simulink subsystem "body_lift_compoenent"  (R2026a)
settings: Solver=VariableStepAuto
settings Model: Creator=joedo  LastModifiedBy=trist

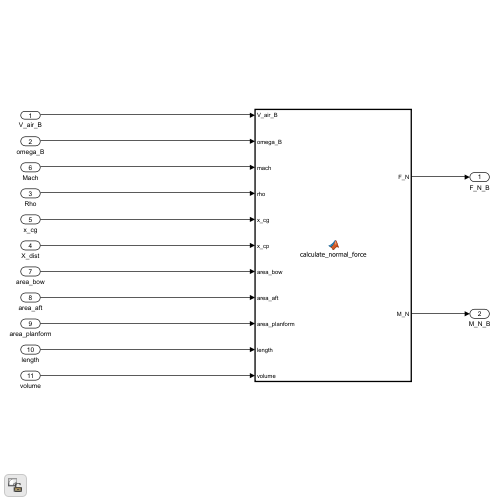
[thumbnail: Simulink's stored preview of the top-level diagram]
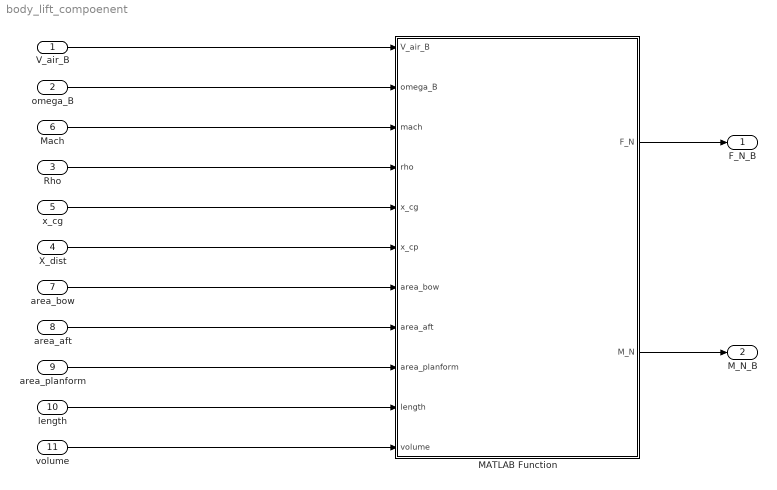
== system body_lift_compoenent ==
  "V_air_B " : Inport
  omega_B : Inport  Port=2
  Rho : Inport  Port=3
  X_dist : Inport  Port=4
  x_cg : Inport  Port=5
  Mach : Inport  Port=6
  area_bow : Inport  Port=7
  area_aft : Inport  Port=8
  area_planform : Inport  Port=9
  length : Inport  Port=10
  volume : Inport  Port=11
  MATLAB Function : MATLAB Function  TreatAsAtomicUnit=on
  F_N_B : Outport  VectorParamsAs1DForOutWhenUnconnected=off
  M_N_B : Outport  Port=2  VectorParamsAs1DForOutWhenUnconnected=off
  wires:
  X_dist/1 -> MATLAB Function/6(x_cp)
  Rho/1 -> MATLAB Function/4(rho)
  "V_air_B "/1 -> MATLAB Function/1(V_air_B)
  omega_B/1 -> MATLAB Function/2(omega_B)
  MATLAB Function/1(F_N) -> F_N_B/1
  MATLAB Function/2(M_N) -> M_N_B/1
  x_cg/1 -> MATLAB Function/5(x_cg)
  Mach/1 -> MATLAB Function/3(mach)
  area_bow/1 -> MATLAB Function/7(area_bow)
  area_aft/1 -> MATLAB Function/8(area_aft)
  area_planform/1 -> MATLAB Function/9(area_planform)
  length/1 -> MATLAB Function/10(length)
  volume/1 -> MATLAB Function/11(volume)

== matlab function body_lift_compoenent/MATLAB Function ==
  data: V_air_B input; omega_B input; mach input; rho input; F_N output; M_N output; x_cg input; x_cp input; area_bow input; area_aft input; area_planform input; length input; volume input
function [F_N, M_N] = calculate_normal_force(V_air_B, omega_B, mach, rho, x_cg, x_cp, area_bow, area_aft, area_planform, length, volume)
    
    lever_arm = [x_cp - x_cg; 0; 0;];

    % relative velocity
    Vrel = V_air_B + cross(omega_B, lever_arm);
    
    % Body relative velocity magnitude
    Vrel_mag = norm(Vrel);
    VrelMagYZ = norm(Vrel(2:3));
    
    if VrelMagYZ ~= 0 % prevent division by 0
        % Angle of attack and component separation
        attack_angle = asin(VrelMagYZ/Vrel_mag);
        F_N_dir = [0; Vrel(2) / VrelMagYZ; Vrel(3) / VrelMagYZ];
        
        % Calculating total force
        [CN, Cm, cp] = aerobody_online(mach, attack_angle, area_bow, area_aft, area_planform, length, volume, x_cp);
        F_N_mag = 0.5 * rho * Vrel_mag^2 * CN;
        F_N = F_N_dir * F_N_mag;
    else
        F_N = [0; 0; 0];
    end
    % Total torque
    M_N = cross(F_N, lever_arm);
end
